simulink model "generateDisturbanceSin"  (R2019a)
settings: Solver=VariableStepAuto  StartTime=0.0  StopTime=tsim  MaxStep=1e-4  RelTol=1e-12  EnableMultiTasking=on
values from neighbouring files (symbols this model uses):
  h = 0.01    [aa_MAGLEV_changeSlope.m]
libraries: cstblocks x1
settings Model: Creator=alcasfra  LastModifiedBy=alcas
settings SolverCC: AlgebraicLoopSolver=LineSearch
settings DataIOCC: ReturnWorkspaceOutputs=off
settings OptimizationCC: LifeSpan=inf
settings DebuggingCC: SFUnexpectedBacktrackingDiag=warning  SFNoUnconditionalDefaultTransitionDiag=warning  ArithmeticOperatorsInVariantConditions=warning
settings SFSimCC: SimUseLocalCustomCode=off
settings RTWCC: RTWUseLocalCustomCode=off
settings CodeAppCC: StateflowObjectComments=on
settings GRTTargetCC: TargetLangStandard=C89/C90 (ANSI)  GeneratePreprocessorConditionals=Disable all
settings ConfigComp: CovMetricSettings=dw  CovHtmlReporting=on  CovSaveCumulativeToWorkspaceVar=on  CovSaveSingleToWorkspaceVar=on  CovExternalEMLEnable=off

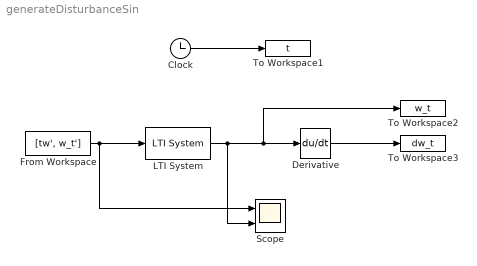
== system generateDisturbanceSin ==
  Clock : Clock
  Derivative : Derivative
  From Workspace : FromWorkspace  VariableName=[tw', w_t']  SampleTime=0
  LTI System : cstblocks/LTI System  sys=filt  IC=[]
  Scope : Scope  NumInputPorts=2
  To Workspace1 : ToWorkspace  VariableName=t  SampleTime=h
      settings: Save2DSignal=2-D array (concatenate along first dimension)
  To Workspace2 : ToWorkspace  VariableName=w_t  SampleTime=h
      settings: Save2DSignal=2-D array (concatenate along first dimension)
  To Workspace3 : ToWorkspace  VariableName=dw_t  SampleTime=h
      settings: Save2DSignal=2-D array (concatenate along first dimension)
  wires:
  Clock/1 -> To Workspace1/1
  Derivative/1 -> To Workspace3/1
  From Workspace/1 -> Scope/1, LTI System/1
  LTI System/1 -> Scope/2, To Workspace2/1, Derivative/1
